simulink model "RectGen"  (R2014b)
settings: Solver=FixedStepDiscrete  SolverMode=SingleTasking  StartTime=0.0  StopTime=20e-6*2  RelTol=1e-3
PreLoadFcn:
  | userName = getenv('UserName');
  | 
  | if strcmp(userName,'Tim')
  | cd C:\MA_1\RectGen
  | else
  | cd D:\MA_1\RectGen
  | end
InitFcn:
  | userName = getenv('UserName');
  | 
  | if strcmp(userName,'Tim')
  | cd C:\MA_1\RectGen
  | else
  | cd D:\MA_1\RectGen
  | end
undefined symbols (not defined in the file): Tb
libraries: xbsIndex_r4 x13
settings Model: Creator=Tim-UML  LastModifiedBy=Tim-UML
settings DebuggingCC: AssertControl=DisableAll
settings HardwareCC: ProdBitPerLong=64  ProdBitPerPointer=64  ProdWordSize=64  ProdHWDeviceType=Generic->64-bit Embedded Processor (LP64)  TargetHWDeviceType=32-bit Generic

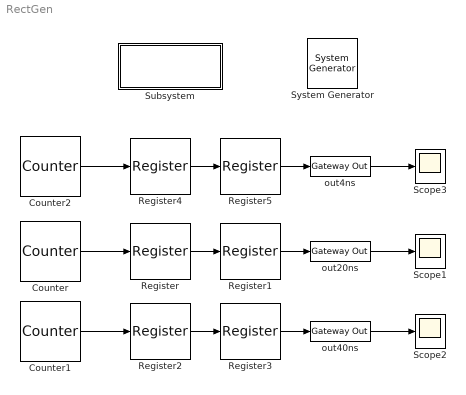
== system RectGen ==
  " System Generator" : xbsIndex_r4/ System Generator  Tag=genX  xilinxfamily=zynq  part=xc7z020  speed=-1  package=clg400  synthesis_tool=Vivado  clock_wrapper=Clock Enables  directory=./netlistFin1  proj_type=Vivado  Synth_file=Vivado Synthesis Defaults  Impl_file=Vivado Implementation Defaults  testbench=on  simulink_period=SystemPeriod  sysclk_period=1000/250  dcm_input_clock_period=10  incr_netlist=off  trim_vbits=Everywhere in SubSystem  dbl_ovrd=According to Block Masks  core_generation=According to Block Masks  run_coregen=off  deprecated_control=off  eval_field=0  block_type=sysgen
  Counter : xbsIndex_r4/Counter  cnt_type=Count Limited  cnt_to=1  operation=Up  start_count=0  cnt_by_val=1  arith_type=Unsigned  n_bits=1  bin_pt=0  load_pin=off  rst=off  en=off  explicit_period=on  period=Tb  use_behavioral_HDL=off  implementation=Fabric  dbl_ovrd=off  block_type=counter
  Counter1 : xbsIndex_r4/Counter  cnt_type=Count Limited  cnt_to=1  operation=Up  start_count=0  cnt_by_val=1  arith_type=Unsigned  n_bits=1  bin_pt=0  load_pin=off  rst=off  en=off  explicit_period=on  period=Tb*2  use_behavioral_HDL=off  implementation=Fabric  dbl_ovrd=off  block_type=counter
  Counter2 : xbsIndex_r4/Counter  cnt_type=Count Limited  cnt_to=1  operation=Up  start_count=0  cnt_by_val=1  arith_type=Unsigned  n_bits=1  bin_pt=0  load_pin=off  rst=off  en=off  explicit_period=on  period=SystemPeriod  use_behavioral_HDL=off  implementation=Fabric  dbl_ovrd=off  block_type=counter
  Register{,1..5} (6 alike) : xbsIndex_r4/Register  init=0  rst=off  en=off  dbl_ovrd=off  block_type=register
  Scope1 : Scope
      settings: TimeRange=1.102458307597285e-07  YMin=-0  YMax=2  SaveName=ScopeData92
  Scope2 : Scope
      settings: TimeRange=1.102458307597285e-07  YMin=-0  YMax=2
  Scope3 : Scope
      settings: TimeRange=1.102458307597285e-07  YMin=-0  YMax=2
  Subsystem : Subsystem  mask(Model Parameters){upsample=No, dmtOfdm=DMT, guardInterval=Yes, AWGN=No, channel=No, equalizer=No, SampleTime=20e-9, BitTime=20e-9, modu_mode=0, radio_precision=fixpoint, bitCount=16, fracLen=13, impulseResponse=No}
      mask prompts: upsample "Enable Upsampling"; dmtOfdm "Select FFT Inputorder"; guardInterval "Guard Interval"; SampleTime "Sample Time [s]"; BitTime "Bit Time"; modu_mode "Modulation Mode"; radio_precision "Select Precision"; bitCount "Bit Count"; fracLen "Fraction Length"; impulseResponse "Measure Impulse Response"
      mask init:
      | initScript
      mask TypeOptions upsample: No | Yes
      mask TypeOptions dmtOfdm: OFDM | DMT
      mask TypeOptions guardInterval: No | Yes
      mask TypeOptions AWGN: No | Yes
      mask TypeOptions channel: No | Yes
      mask TypeOptions equalizer: No | Yes
      mask TypeOptions radio_precision: double | fixpoint
      mask TypeOptions impulseResponse: No | Yes
      mask DialogControl Container3 Prompt: Only for Fixpoint
      mask Display: disp('Edit Model\n Parameters')
  out20ns : xbsIndex_r4/Gateway Out  inherit_from_input=on  hdl_port=on  rows=1  columns=1  UseAsDAC=off  DACChannel='1'  interface=None  automatic_assignment=on  address_offset=hex2dec('00')  intf_description=''  timing_constraint=None  locs_specified=off  LOCs={}  io_standard={}  block_type=gatewayout
  out40ns : xbsIndex_r4/Gateway Out  inherit_from_input=on  hdl_port=on  rows=1  columns=1  UseAsDAC=off  DACChannel='1'  interface=None  automatic_assignment=on  address_offset=hex2dec('00')  intf_description=''  timing_constraint=None  locs_specified=off  LOCs={}  io_standard={}  block_type=gatewayout
  out4ns : xbsIndex_r4/Gateway Out  inherit_from_input=on  hdl_port=on  rows=1  columns=1  UseAsDAC=off  DACChannel='1'  interface=None  automatic_assignment=on  address_offset=hex2dec('00')  intf_description=''  timing_constraint=None  locs_specified=off  LOCs={}  io_standard={}  block_type=gatewayout
  wires:
  out20ns/1 -> Scope1/1
  Register/1 -> Register1/1
  Register1/1 -> out20ns/1
  Counter/1 -> Register/1
  out40ns/1 -> Scope2/1
  Register2/1 -> Register3/1
  Register3/1 -> out40ns/1
  Counter1/1 -> Register2/1
  out4ns/1 -> Scope3/1
  Register4/1 -> Register5/1
  Register5/1 -> out4ns/1
  Counter2/1 -> Register4/1

== system RectGen/Subsystem ==
